simulink model "untitled"  (R2023a)
settings: Solver=VariableStepAuto  StartTime=0.0  StopTime=10  RelTol=1e-3
libraries: simulink x4
settings Model: Creator=yaros  LastModifiedBy=yaros

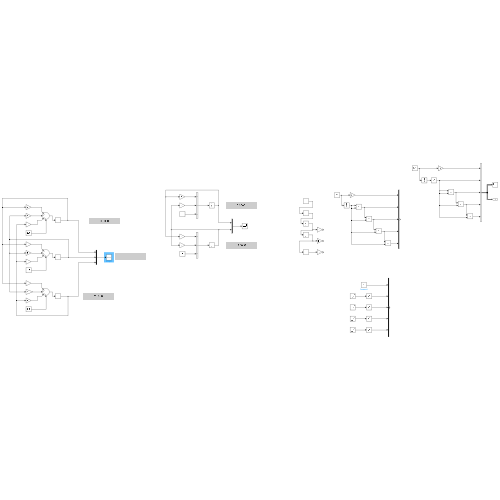
[thumbnail: Simulink's stored preview of the top-level diagram]
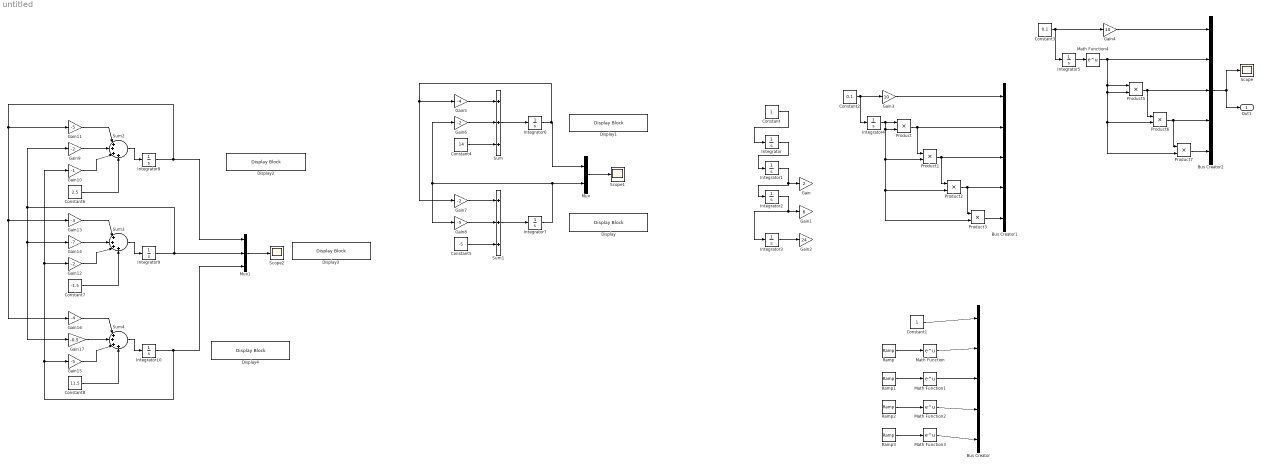
== system untitled ==
  Bus Creator : BusCreator  Inputs=5
  Bus Creator1 : BusCreator  Inputs=5
  Bus Creator2 : BusCreator  Inputs=5
  Constant : Constant
  Constant1 : Constant
  Constant2 : Constant  Value=0.1
  Constant3 : Constant  Value=0.1
  Constant4 : Constant  Value=14
  Constant5 : Constant  Value=-5
  Constant6 : Constant  Value=2.5
  Constant7 : Constant  Value=-1.5
  Constant8 : Constant  Value=11.5
  Display{,1..4} (5 alike) : DisplayBlock  LabelPosition=Hide  Transparency=1
  Gain : Gain  Gain=2
  Gain1 : Gain  Gain=6
  Gain10 : Gain  Gain=-1
  Gain11 : Gain  Gain=-5
  Gain{6..7,9,12} (4 alike) : Gain  Gain=-2
  Gain13 : Gain  Gain=-3
  Gain14 : Gain  Gain=-7
  Gain15 : Gain  Gain=-5
  Gain16 : Gain  Gain=-4
  Gain17 : Gain  Gain=-0.5
  Gain2 : Gain  Gain=24
  Gain3 : Gain  Gain=10
  Gain4 : Gain  Gain=10
  Gain5 : Gain  Gain=-4
  Gain8 : Gain  Gain=-5
  Integrator{,1..10} (11 alike) : Integrator
  Math Function{,1..4} (5 alike) : Math
  Mux : Mux  Inputs=2
  Mux1 : Mux  Inputs=3
  Product{,1..3,5..7} (7 alike) : Product
  Ramp : simulink/Sources/Ramp  slope=1  start=0  InitialOutput=0
  Ramp1 : simulink/Sources/Ramp  slope=2  start=0  InitialOutput=0
  Ramp2 : simulink/Sources/Ramp  slope=4  start=0  InitialOutput=0
  Ramp3 : simulink/Sources/Ramp  slope=16  start=0  InitialOutput=0
  Scope : Scope
  Scope1 : Scope
  Scope2 : Scope
  Sum : Sum  Inputs=+++
  Sum1 : Sum  Inputs=+++
  Sum2 : Sum  Inputs=|++++
  Sum3 : Sum  Inputs=|++++
  Sum4 : Sum  Inputs=|++++
  Out1 : Outport
  wires:
  Constant/1 -> Integrator/1
  Integrator/1 -> Integrator1/1
  Integrator1/1 -> Integrator2/1, Gain/1
  Integrator2/1 -> Gain1/1, Integrator3/1
  Integrator3/1 -> Gain2/1
  Constant1/1 -> Bus Creator/1
  Ramp/1 -> Math Function/1
  Math Function/1 -> Bus Creator/2
  Ramp1/1 -> Math Function1/1
  Math Function1/1 -> Bus Creator/3
  Ramp2/1 -> Math Function2/1
  Math Function2/1 -> Bus Creator/4
  Ramp3/1 -> Math Function3/1
  Math Function3/1 -> Bus Creator/5
  Constant2/1 -> Integrator4/1, Gain3/1
  Gain3/1 -> Bus Creator1/1
  Integrator4/1 -> Product/2, Product1/2, Product2/2, Product3/2, Product/1
  Product/1 -> Product1/1, Bus Creator1/2
  Product1/1 -> Product2/1, Bus Creator1/3
  Product2/1 -> Product3/1, Bus Creator1/4
  Product3/1 -> Bus Creator1/5
  Math Function4/1 -> Bus Creator2/2, Product5/1, Product5/2, Product6/2, Product7/2
  Gain4/1 -> Bus Creator2/1
  Product5/1 -> Product6/1, Bus Creator2/3
  Product6/1 -> Product7/1, Bus Creator2/4
  Constant3/1 -> Integrator5/1, Gain4/1
  Product7/1 -> Bus Creator2/5
  Bus Creator2/1 -> Out1/1, Scope/1
  Integrator5/1 -> Math Function4/1
  Gain5/1 -> Sum/1
  Gain6/1 -> Sum/2
  Constant4/1 -> Sum/3
  Sum/1 -> Integrator6/1
  Sum1/1 -> Integrator7/1
  Gain8/1 -> Sum1/2
  Gain7/1 -> Sum1/1
  Constant5/1 -> Sum1/3
  Integrator6/1 -> Gain5/1, Gain7/1, Mux/1
  Mux/1 -> Scope1/1
  Integrator7/1 -> Mux/2, Gain6/1, Gain8/1
  Sum2/1 -> Integrator8/1
  Constant6/1 -> Sum2/4
  Gain10/1 -> Sum2/3
  Gain9/1 -> Sum2/2
  Gain11/1 -> Sum2/1
  Gain12/1 -> Sum3/3
  Gain13/1 -> Sum3/1
  Sum3/1 -> Integrator9/1
  Constant7/1 -> Sum3/4
  Gain14/1 -> Sum3/2
  Gain15/1 -> Sum4/3
  Gain16/1 -> Sum4/1
  Sum4/1 -> Integrator10/1
  Constant8/1 -> Sum4/4
  Gain17/1 -> Sum4/2
  Mux1/1 -> Scope2/1
  Integrator8/1 -> Gain13/1, Gain16/1, Gain11/1, Mux1/1
  Integrator9/1 -> Gain14/1, Gain17/1, Gain9/1, Mux1/2
  Integrator10/1 -> Gain12/1, Gain10/1, Gain15/1, Mux1/3
